simulink model "slb_tunable_param"  (R2015b)
settings: Solver=FixedStepDiscrete  SolverMode=SingleTasking  StartTime=0.0  StopTime=10.0  RelTol=1e-3
libraries: simulink x1
settings Model: Creator=amatsumo  LastModifiedBy=amatsumo
settings DataIOCC: SaveFormat=Array  SignalLoggingSaveFormat=ModelDataLogs  SaveOutput=off  SignalLogging=off  SaveTime=off
settings OptimizationCC: BlockReduction=off  ConditionallyExecuteInputs=off  DefaultParameterBehavior=Inlined  ExpressionDepthLimit=2147483647
settings DebuggingCC: AlgebraicLoopMsg=error  UnderspecifiedInitializationDetection=Classic  MergeDetectMultiDrivingBlocksExec=none  SolverPrmCheckMsg=warning  InheritedTsInSrcMsg=none  SingleTaskRateTransMsg=error  FcnCallInpInsideContextMsg=EnableAllAsWarning  StateNameClashWarn=warning
settings HardwareCC: ProdBitPerPointer=32  ProdLargestAtomicFloat=None  ProdIntDivRoundTo=Undefined  ProdEndianess=Unspecified  ProdWordSize=32  ProdHWDeviceType=ASIC/FPGA->ASIC/FPGA  ProdEqTarget=off
settings GRTTargetCC: GeneratePreprocessorConditionals=Disable all  CombineOutputUpdateFcns=off  GRTInterface=on
settings ConfigComp: CovModelRefEnable=Off  CovSFcnEnable=off

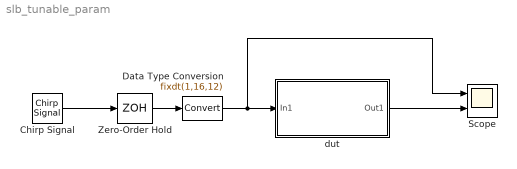
== system slb_tunable_param ==
  Chirp Signal : simulink/Sources/Chirp Signal  f1=10  T=10  f2=500
  Data Type Conversion : DataTypeConversion  OutDataTypeStr=fixdt(1,16,12)
  Scope : Scope  NumInputPorts=2
  Zero-Order Hold : ZeroOrderHold  SampleTime=1/1000
  dut : Subsystem
  wires:
  Chirp Signal/1 -> Zero-Order Hold/1
  Zero-Order Hold/1 -> Data Type Conversion/1
  dut/1(Out1) -> Scope/2
  Data Type Conversion/1 -> Scope/1, dut/1(In1)

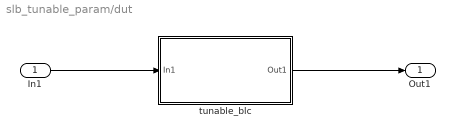
== system slb_tunable_param/dut ==
  In1 : Inport
  tunable_blc : Subsystem  TreatAsAtomicUnit=on  mask{a1=1.5, a2=2.2, c1=3}
      mask prompts: a1 "Gain1"; a2 "Gain2"; c1 "Constant"
  Out1 : Outport
  wires:
  In1/1 -> tunable_blc/1(In1)
  tunable_blc/1(Out1) -> Out1/1

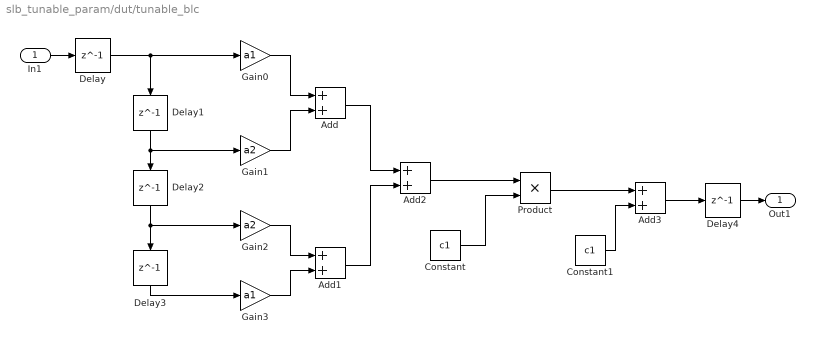
== system slb_tunable_param/dut/tunable_blc ==
  In1 : Inport
  Add{,1..3} (4 alike) : Sum
  Constant : Constant  Value=c1  OutDataTypeStr=fixdt(1,16,12)
  Constant1 : Constant  Value=c1  OutDataTypeStr=fixdt(1,16,12)
  Delay{,1..4} (5 alike) : Delay  DelayLength=1
  Gain0 : Gain  Gain=a1  ParamDataTypeStr=fixdt(1,16,12)  OutDataTypeStr=Inherit: Same as input
  Gain1 : Gain  Gain=a2  ParamDataTypeStr=fixdt(1,16,12)  OutDataTypeStr=Inherit: Same as input
  Gain2 : Gain  Gain=a2  ParamDataTypeStr=fixdt(1,16,12)  OutDataTypeStr=Inherit: Same as input
  Gain3 : Gain  Gain=a1  ParamDataTypeStr=fixdt(1,16,12)  OutDataTypeStr=Inherit: Same as input
  Product : Product  RndMeth=Zero
  Out1 : Outport
  wires:
  Delay/1 -> Delay1/1, Gain0/1
  Delay1/1 -> Delay2/1, Gain1/1
  Delay2/1 -> Delay3/1, Gain2/1
  Gain0/1 -> Add/1
  Gain1/1 -> Add/2
  Gain2/1 -> Add1/1
  Gain3/1 -> Add1/2
  Add/1 -> Add2/1
  Add1/1 -> Add2/2
  Add2/1 -> Product/1
  Constant/1 -> Product/2
  Delay3/1 -> Gain3/1
  In1/1 -> Delay/1
  Delay4/1 -> Out1/1
  Product/1 -> Add3/1
  Add3/1 -> Delay4/1
  Constant1/1 -> Add3/2
